simulink model "pidLoopTest"  (R2017a)
settings: Solver=VariableStepAuto  StartTime=0.0  StopTime=10  RelTol=1e-3
undefined symbols (not defined in the file or in its folder): fpgaClk, PWMFreq
libraries: simulink x2
settings Model: Creator=Nicoe Welch  LastModifiedBy=Nicoe Welch

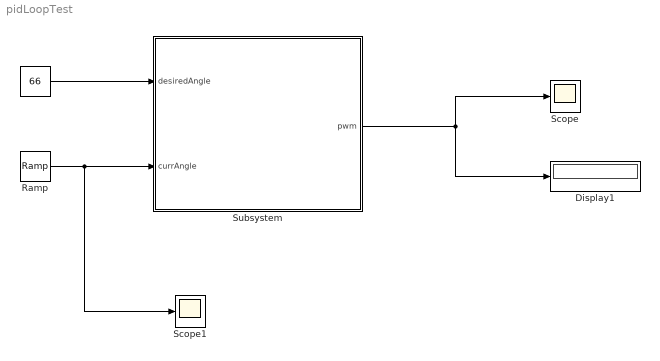
== system pidLoopTest ==
  " " : Constant  Value=66
  Display1 : Display
  Ramp : simulink/Sources/Ramp  slope=1  start=0  X0=60
  Scope : Scope
  Scope1 : Scope
  Subsystem : Subsystem
  wires:
  Subsystem/1(pwm) -> Display1/1, Scope/1
  Ramp/1 -> Scope1/1, Subsystem/2(currAngle)
  " "/1 -> Subsystem/1(desiredAngle)

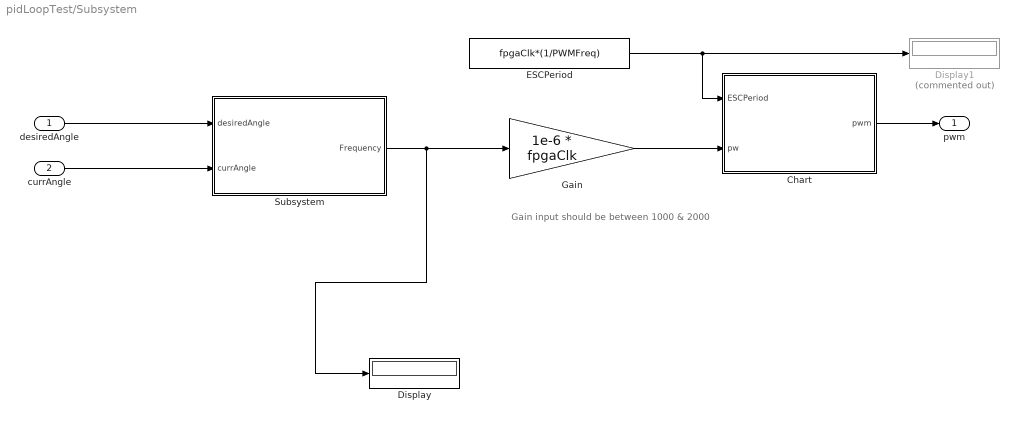
== system pidLoopTest/Subsystem ==
  note: Gain input should be between 1000 & 2000
  desiredAngle : Inport
  currAngle : Inport  Port=2
  Chart : Stateflow chart  TreatAsAtomicUnit=on
  Display : Display
  Display1 : Display  Commented=on
  ESCPeriod : Constant  Value=fpgaClk*(1/PWMFreq)  OutDataTypeStr=uint32
  Gain : Gain  Gain=1e-6 * fpgaClk  OutDataTypeStr=Inherit: Same as input
  Subsystem : Subsystem
  pwm : Outport
  wires:
  Gain/1 -> Chart/2(pw)
  ESCPeriod/1 -> Chart/1(ESCPeriod), Display1/1
  Chart/1(pwm) -> pwm/1
  desiredAngle/1 -> Subsystem/1(desiredAngle)
  currAngle/1 -> Subsystem/2(currAngle)
  Subsystem/1(Frequency) -> Display/1, Gain/1

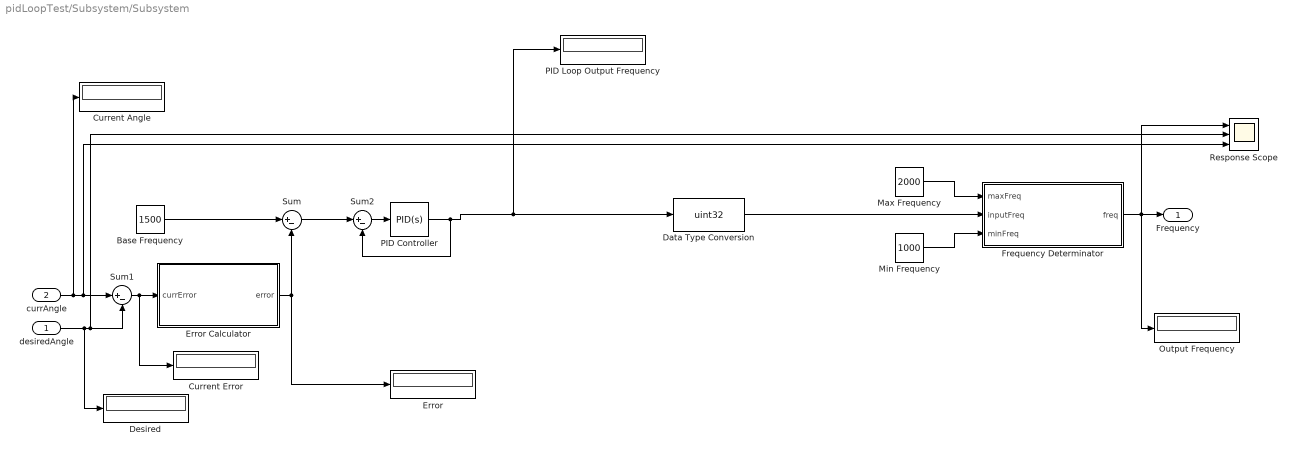
== system pidLoopTest/Subsystem/Subsystem ==
  desiredAngle : Inport
  currAngle : Inport  Port=2
  Base Frequency : Constant  Value=1500
  Current Angle : Display
  Current Error : Display
  Data Type Conversion : DataTypeConversion  OutDataTypeStr=uint32  RndMeth=Nearest
  Desired : Display
  Error : Display
  Error Calculator : MATLAB Function  TreatAsAtomicUnit=on
  Frequency Determinator : MATLAB Function  TreatAsAtomicUnit=on
  Max Frequency : Constant  Value=2000  OutDataTypeStr=uint32
  Min Frequency : Constant  Value=1000  OutDataTypeStr=uint32
  Output Frequency : Display
  PID Controller : simulink/Continuous/PID Controller  Controller=PID  TimeDomain=Continuous-time  SampleTime=-1  IntegratorMethod=Forward Euler  FilterMethod=Forward Euler  Form=Parallel  UseFilter=on  ControllerParametersSource=internal  P=0  I=1  D=0  N=100  InitialConditionSource=internal  InitialConditionForIntegrator=0  InitialConditionForFilter=0  ExternalReset=none  LimitOutput=off  UpperSaturationLimit=inf  LowerSaturationLimit=-inf  LinearizeAsGain=on  AntiWindupMode=none  Kb=1  TrackingMode=off  Kt=1  PParamMin=[]  PParamMax=[]  IParamMin=[]  IParamMax=[]  DParamMin=[]  DParamMax=[]  NParamMin=[]  NParamMax=[]  KbParamMin=[]  KbParamMax=[]  KtParamMin=[]  KtParamMax=[]  POutMin=[]  POutMax=[]  IOutMin=[]  IOutMax=[]  DOutMin=[]  DOutMax=[]  NOutMin=[]  NOutMax=[]  KbOutMin=[]  KbOutMax=[]  KtOutMin=[]  KtOutMax=[]  IntegratorOutMin=[]  IntegratorOutMax=[]  FilterOutMin=[]  FilterOutMax=[]  SumOutMin=[]  SumOutMax=[]  SumI1OutMin=[]  SumI1OutMax=[]  SumI2OutMin=[]  SumI2OutMax=[]  SumI3OutMin=[]  SumI3OutMax=[]  SumDOutMin=[]  SumDOutMax=[]  SaturationOutMin=[]  SaturationOutMax=[]  IntegratorContinuousStateAttributes=''  IntegratorStateMustResolveToSignalObject=off  IntegratorRTWStateStorageClass=Auto  FilterContinuousStateAttributes=''  FilterStateMustResolveToSignalObject=off  FilterRTWStateStorageClass=Auto  DifferentiatorICPrevScaledInput=0  DifferentiatorOutMin=[]  DifferentiatorOutMax=[]  InitialConditionSetting=State (most efficient)
  PID Loop Output Frequency : Display
  Response Scope : Scope  NumInputPorts=3
  Sum : Sum  Inputs=|+-
  Sum1 : Sum  Inputs=|+-
  Sum2 : Sum  Inputs=|+-
  Frequency : Outport
  wires:
  Base Frequency/1 -> Sum/1
  Frequency Determinator/1(freq) -> Response Scope/1, Output Frequency/1, Frequency/1
  Min Frequency/1 -> Frequency Determinator/3(minFreq)
  Max Frequency/1 -> Frequency Determinator/1(maxFreq)
  desiredAngle/1 -> Desired/1, Sum1/2, Response Scope/2
  currAngle/1 -> Current Angle/1, Sum1/1, Response Scope/3
  Error Calculator/1(error) -> Error/1, Sum/2
  Sum1/1 -> Current Error/1, Error Calculator/1(currError)
  Data Type Conversion/1 -> Frequency Determinator/2(inputFreq)
  Sum/1 -> Sum2/1
  Sum2/1 -> PID Controller/1
  PID Controller/1 -> Data Type Conversion/1, PID Loop Output Frequency/1, Sum2/2

== stateflow chart pidLoopTest/Subsystem/Chart ==
  settings: executeAtInitialization=1
  state on
    entry: cnt = uint32(0);
    pwm = true;
    during: cnt = cnt + 1;
  state off
    entry: pwm = false;
    during: cnt = cnt + 1;
  (default) -> on
  on -> off : [cnt > pw]
  off -> on : [cnt >= ESCPeriod]
  data: ESCPeriod input uint32; pw input uint32; pwm output boolean; cnt local uint32

== matlab function pidLoopTest/Subsystem/Subsystem/Error Calculator ==
  data: error output; currError input
function error = fcn(currError)
if currError < 40 && currError > -40
    transError = -.01080*(currError)^3 + .678*(currError)^2 + 2.124*(currError) + 22.653;
else
    if currError > 40
        transError = 500;
    else
        transError = -500;
    end
end

if currError < 0
    error = transError * -1;
elseif currError == 0
    error = currError;
else
    error = transError;
end

== matlab function pidLoopTest/Subsystem/Subsystem/Frequency Determinator ==
  data: maxFreq input; inputFreq input; freq output uint32; minFreq input
function freq = fcn(maxFreq,inputFreq, minFreq)
    if( inputFreq > maxFreq ) 
        freq = maxFreq
    elseif ( inputFreq < minFreq ) 
        freq = minFreq
    else 
        freq = inputFreq
    end
